simulink model "Example_Pendulum"  (R2017a)
settings: Solver=VariableStepAuto  StartTime=0.0  StopTime=10.0  RelTol=1e-3
settings Model: Creator=lerch  LastModifiedBy=lerch
settings OptimizationCC: DefaultParameterBehavior=Inlined

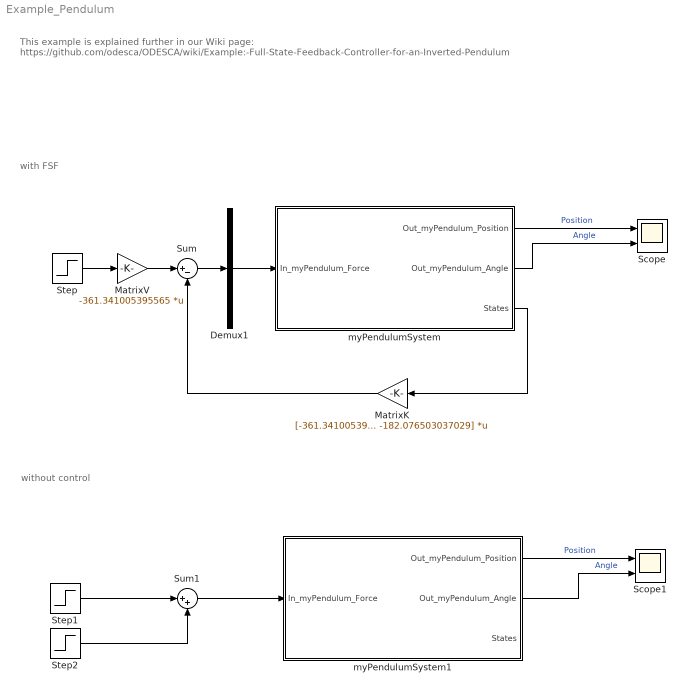
== system Example_Pendulum ==
  note: without control
  note: with FSF
  note: This example is explained further in our Wiki page:
      | https://github.com/odesca/ODESCA/wiki/Example:-Full-State-Feedback-Controller-for-an-Inverted-Pendulum
  Demux1 : Demux  Outputs=1
  MatrixK : Gain  Gain=[-361.341005395564 -250.256467562303 -795.986015606006 -182.076503037029]  Multiplication=Matrix(K*u)
  MatrixV : Gain  Gain=-361.341005395565  Multiplication=Matrix(K*u)
  Scope : Scope  NumInputPorts=2
  Scope1 : Scope  NumInputPorts=2
  Step : Step  SampleTime=0
  Step1 : Step  After=0.2  SampleTime=0
  Step2 : Step  Time=1.5  After=-0.2  SampleTime=0
  Sum : Sum  Inputs=|+-
  Sum1 : Sum  Inputs=|++
  myPendulumSystem : Subsystem  mask(myPendulumSystem){initState=[0,0,0,0], myPendulum_M0=4, myPendulum_M1=0.36, myPendulum_l_s=0.451, myPendulum_theta=0.08433, myPendulum_Fr=10, myPendulum_C=0.00145, myPendulum_g=9.81}
      mask prompts: initState "Initial State is a column vector of 4 elements:

x1 = myPendulum_Position [m]
x2 = myPendulum_Velocity [m/s]
x3 = myPendulum_Angle [rad]
x4 = myPendulum_AngularSpeed [rad/s]

Initial State:"; myPendulum_M0 "M0
[kg]"; myPendulum_M1 "M1
[kg]"; myPendulum_l_s "l_s
[m]"; myPendulum_theta "theta
[kgm^2]"; myPendulum_Fr "Fr
[kg/s]"; myPendulum_C "C
[kgm^2/s]"; myPendulum_g "g
[m/s^2]"
      mask help:
      | This system consists of:
      |
      | 1 Components
      | 4 States
      | 1 Inputs
      | 2 Outputs
      | 7 Parameters
  myPendulumSystem1 : Subsystem  mask(myPendulumSystem){initState=[0,0,0,0], myPendulum_M0=4, myPendulum_M1=0.36, myPendulum_l_s=0.451, myPendulum_theta=0.08433, myPendulum_Fr=10, myPendulum_C=0.00145, myPendulum_g=9.81}
      mask prompts: initState "Initial State is a column vector of 4 elements:

x1 = myPendulum_Position [m]
x2 = myPendulum_Velocity [m/s]
x3 = myPendulum_Angle [rad]
x4 = myPendulum_AngularSpeed [rad/s]

Initial State:"; myPendulum_M0 "M0
[kg]"; myPendulum_M1 "M1
[kg]"; myPendulum_l_s "l_s
[m]"; myPendulum_theta "theta
[kgm^2]"; myPendulum_Fr "Fr
[kg/s]"; myPendulum_C "C
[kgm^2/s]"; myPendulum_g "g
[m/s^2]"
      mask help:
      | This system consists of:
      |
      | 1 Components
      | 4 States
      | 1 Inputs
      | 2 Outputs
      | 7 Parameters
  wires:
  myPendulumSystem/3(States) -> MatrixK/1
  Demux1/1 -> myPendulumSystem/1(In_myPendulum_Force)
  MatrixK/1 -> Sum/2
  Step/1 -> MatrixV/1
  Sum/1 -> Demux1/1
  myPendulumSystem/1(Out_myPendulum_Position) -> Scope/1  "Position"
  myPendulumSystem/2(Out_myPendulum_Angle) -> Scope/2  "Angle"
  MatrixV/1 -> Sum/1
  Sum1/1 -> myPendulumSystem1/1(In_myPendulum_Force)
  Step1/1 -> Sum1/1
  Step2/1 -> Sum1/2
  myPendulumSystem1/1(Out_myPendulum_Position) -> Scope1/1  "Position"
  myPendulumSystem1/2(Out_myPendulum_Angle) -> Scope1/2  "Angle"

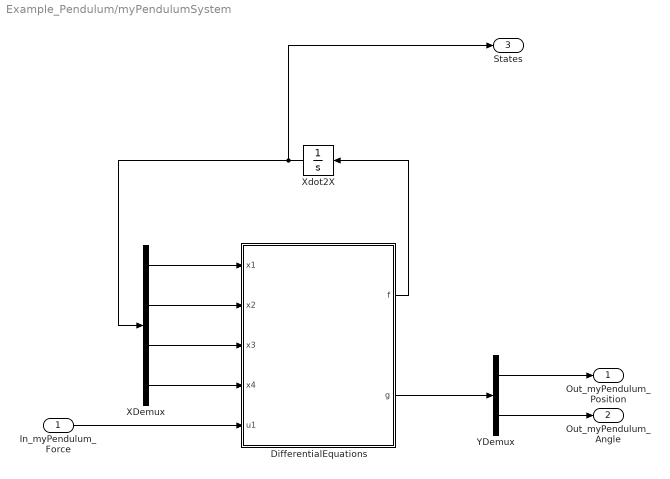
== system Example_Pendulum/myPendulumSystem ==
  In_myPendulum_Force : Inport
  DifferentialEquations : MATLAB Function  TreatAsAtomicUnit=on
  XDemux : Demux
  Xdot2X : Integrator  InitialCondition=initState
  YDemux : Demux  Outputs=2
  Out_myPendulum_Position : Outport
  Out_myPendulum_Angle : Outport  Port=2
  States : Outport  Port=3
  wires:
  In_myPendulum_Force/1 -> DifferentialEquations/5(u1)
  DifferentialEquations/2(g) -> YDemux/1
  YDemux/1 -> Out_myPendulum_Position/1
  YDemux/2 -> Out_myPendulum_Angle/1
  XDemux/1 -> DifferentialEquations/1(x1)
  XDemux/2 -> DifferentialEquations/2(x2)
  XDemux/3 -> DifferentialEquations/3(x3)
  XDemux/4 -> DifferentialEquations/4(x4)
  DifferentialEquations/1(f) -> Xdot2X/1
  Xdot2X/1 -> XDemux/1, States/1

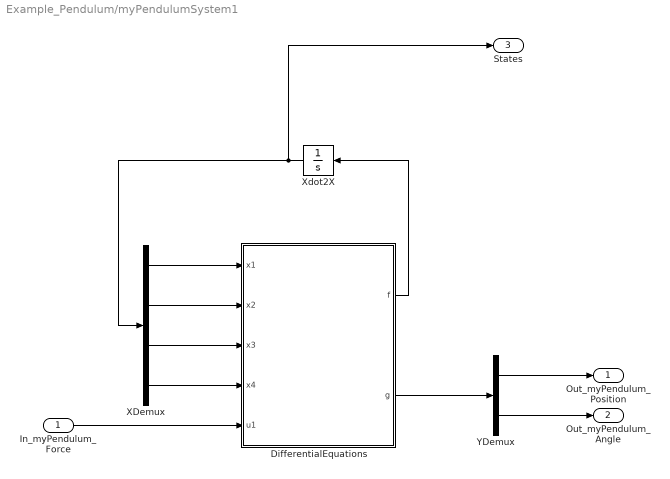
== system Example_Pendulum/myPendulumSystem1 ==
  In_myPendulum_Force : Inport
  DifferentialEquations : MATLAB Function  TreatAsAtomicUnit=on
  XDemux : Demux
  Xdot2X : Integrator  InitialCondition=initState
  YDemux : Demux  Outputs=2
  Out_myPendulum_Position : Outport
  Out_myPendulum_Angle : Outport  Port=2
  States : Outport  Port=3
  wires:
  Xdot2X/1 -> States/1, XDemux/1
  DifferentialEquations/1(f) -> Xdot2X/1
  XDemux/4 -> DifferentialEquations/4(x4)
  XDemux/3 -> DifferentialEquations/3(x3)
  XDemux/2 -> DifferentialEquations/2(x2)
  XDemux/1 -> DifferentialEquations/1(x1)
  YDemux/2 -> Out_myPendulum_Angle/1
  YDemux/1 -> Out_myPendulum_Position/1
  DifferentialEquations/2(g) -> YDemux/1
  In_myPendulum_Force/1 -> DifferentialEquations/5(u1)

== matlab function Example_Pendulum/myPendulumSystem1/DifferentialEquations ==
  data: x1 input; f output; x2 input; x3 input; x4 input; u1 input; g output; myPendulum_g parameter; myPendulum_C parameter; myPendulum_Fr parameter; myPendulum_theta parameter; myPendulum_l_s parameter; myPendulum_M1 parameter; myPendulum_M0 parameter
function [f,g] = DifferentialEquations(x1,x2,x3,x4,u1,myPendulum_g, myPendulum_C, myPendulum_Fr, myPendulum_theta, myPendulum_l_s, myPendulum_M1, myPendulum_M0)
%#codegen

%    This function was generated by the Symbolic Math Toolbox version 7.2.
%    06-Sep-2019 13:49:40

t2 = sin(x3);
t3 = myPendulum_M1.^2;
t4 = myPendulum_l_s.^2;
t5 = myPendulum_M0+myPendulum_M1;
t6 = myPendulum_theta.*t5;
t9 = t3.*t4;
t7 = t6-t9;
t8 = 1.0./t7;
t10 = cos(x3);
t11 = t2.^2;
t12 = t3.*t4.*t8.*t11;
t13 = t12+1.0;
t14 = 1.0./t13;
t15 = x4.^2;
f = [x2;t14.*(myPendulum_theta.*t8.*u1-myPendulum_Fr.*myPendulum_theta.*t8.*x2+myPendulum_M1.*myPendulum_l_s.*myPendulum_theta.*t2.*t8.*t15+myPendulum_C.*myPendulum_M1.*myPendulum_l_s.*t8.*t10.*x4-myPendulum_g.*t2.*t3.*t4.*t8.*t10);x4;-t14.*(myPendulum_C.*t5.*t8.*x4+myPendulum_M1.*myPendulum_l_s.*t8.*t10.*u1-myPendulum_M1.*myPendulum_g.*myPendulum_l_s.*t2.*t5.*t8-myPendulum_M1.*myPendulum_Fr.*myPendulum_l_s.*t8.*t10.*x2+t2.*t3.*t4.*t8.*t10.*t15)];
if nargout > 1
    g = [x1;x3];
end

== matlab function Example_Pendulum/myPendulumSystem/DifferentialEquations ==
  data: x1 input; f output; x2 input; x3 input; x4 input; u1 input; g output; myPendulum_g parameter; myPendulum_C parameter; myPendulum_Fr parameter; myPendulum_theta parameter; myPendulum_l_s parameter; myPendulum_M1 parameter; myPendulum_M0 parameter
function [f,g] = DifferentialEquations(x1,x2,x3,x4,u1,myPendulum_g, myPendulum_C, myPendulum_Fr, myPendulum_theta, myPendulum_l_s, myPendulum_M1, myPendulum_M0)
%#codegen

%    This function was generated by the Symbolic Math Toolbox version 7.2.
%    06-Sep-2019 13:49:40

t2 = sin(x3);
t3 = myPendulum_M1.^2;
t4 = myPendulum_l_s.^2;
t5 = myPendulum_M0+myPendulum_M1;
t6 = myPendulum_theta.*t5;
t9 = t3.*t4;
t7 = t6-t9;
t8 = 1.0./t7;
t10 = cos(x3);
t11 = t2.^2;
t12 = t3.*t4.*t8.*t11;
t13 = t12+1.0;
t14 = 1.0./t13;
t15 = x4.^2;
f = [x2;t14.*(myPendulum_theta.*t8.*u1-myPendulum_Fr.*myPendulum_theta.*t8.*x2+myPendulum_M1.*myPendulum_l_s.*myPendulum_theta.*t2.*t8.*t15+myPendulum_C.*myPendulum_M1.*myPendulum_l_s.*t8.*t10.*x4-myPendulum_g.*t2.*t3.*t4.*t8.*t10);x4;-t14.*(myPendulum_C.*t5.*t8.*x4+myPendulum_M1.*myPendulum_l_s.*t8.*t10.*u1-myPendulum_M1.*myPendulum_g.*myPendulum_l_s.*t2.*t5.*t8-myPendulum_M1.*myPendulum_Fr.*myPendulum_l_s.*t8.*t10.*x2+t2.*t3.*t4.*t8.*t10.*t15)];
if nargout > 1
    g = [x1;x3];
end
